simulink model "Automotive_model2"  (R2020b)
settings: Solver=VariableStepAuto  StartTime=0.0  StopTime=97  RelTol=1e-3
undefined symbols (not defined in the file): sigbuilder_block
libraries: simulink x23
(part 2 of 2)

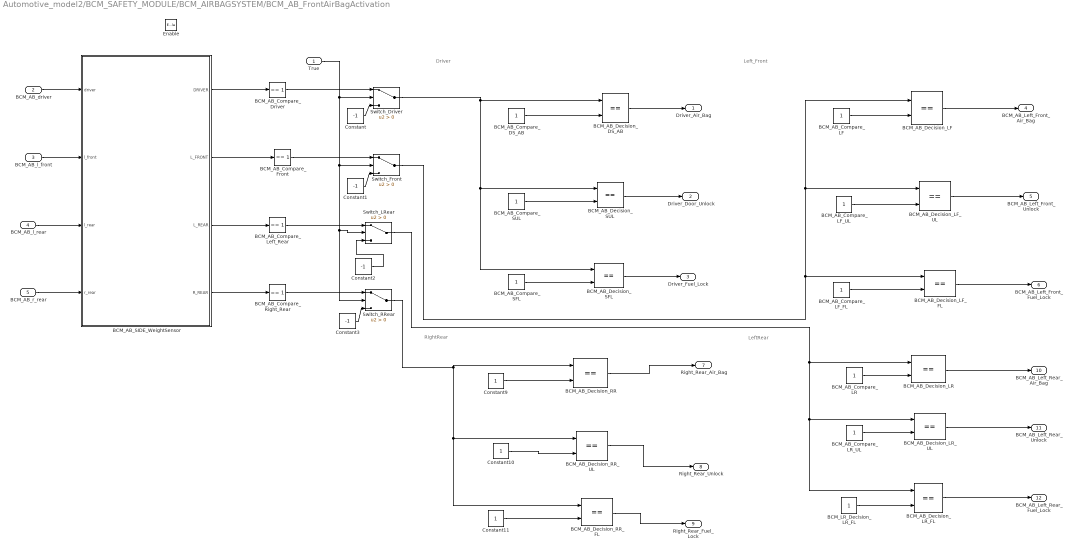
== system Automotive_model2/BCM_SAFETY_MODULE/BCM_AIRBAGSYSTEM/BCM_AB_FrontAirBagActivation ==
  note: RightRear
  note: LeftRear
  note: Left_Front
  note: Driver
  True : Inport
  BCM_AB_driver : Inport  Port=2
  BCM_AB_l_front : Inport  Port=3
  BCM_AB_l_rear : Inport  Port=4
  BCM_AB_r_rear : Inport  Port=5
  Enable : EnablePort
  BCM_AB_Compare_DS_AB : Constant
  BCM_AB_Compare_Driver : simulink/Logic and Bit Operations/Compare To Constant  relop===  const=1  OutDataTypeStr=boolean
  BCM_AB_Compare_Front : simulink/Logic and Bit Operations/Compare To Constant  relop===  const=1  OutDataTypeStr=boolean
  BCM_AB_Compare_LF : Constant
  BCM_AB_Compare_LF_FL : Constant
  BCM_AB_Compare_LF_UL : Constant
  BCM_AB_Compare_LR : Constant
  BCM_AB_Compare_LR_UL : Constant
  BCM_AB_Compare_Left_Rear : simulink/Logic and Bit Operations/Compare To Constant  relop===  const=1  OutDataTypeStr=boolean
  BCM_AB_Compare_Right_Rear : simulink/Logic and Bit Operations/Compare To Constant  relop===  const=1  OutDataTypeStr=boolean
  BCM_AB_Compare_SFL : Constant
  BCM_AB_Compare_SUL : Constant
  BCM_AB_Decision_DS_AB : RelationalOperator  Operator===  OutDataTypeStr=boolean  RndMeth=Simplest
  BCM_AB_Decision_LF : RelationalOperator  Operator===  OutDataTypeStr=boolean  RndMeth=Simplest
  BCM_AB_Decision_LF_FL : RelationalOperator  Operator===  OutDataTypeStr=boolean  RndMeth=Simplest
  BCM_AB_Decision_LF_UL : RelationalOperator  Operator===  OutDataTypeStr=boolean  RndMeth=Simplest
  BCM_AB_Decision_LR : RelationalOperator  Operator===  OutDataTypeStr=boolean  RndMeth=Simplest
  BCM_AB_Decision_LR_FL : RelationalOperator  Operator===  OutDataTypeStr=boolean  RndMeth=Simplest
  BCM_AB_Decision_LR_UL : RelationalOperator  Operator===  OutDataTypeStr=boolean  RndMeth=Simplest
  BCM_AB_Decision_RR : RelationalOperator  Operator===  OutDataTypeStr=boolean  RndMeth=Simplest
  BCM_AB_Decision_RR_FL : RelationalOperator  Operator===  OutDataTypeStr=boolean  RndMeth=Simplest
  BCM_AB_Decision_RR_UL : RelationalOperator  Operator===  OutDataTypeStr=boolean  RndMeth=Simplest
  BCM_AB_Decision_SFL : RelationalOperator  Operator===  OutDataTypeStr=boolean  RndMeth=Simplest
  BCM_AB_Decision_SUL : RelationalOperator  Operator===  OutDataTypeStr=boolean  RndMeth=Simplest
  BCM_AB_SIDE_WeightSensor : MATLAB Function  TreatAsAtomicUnit=on
  BCM_LR_Decision_LR_FL : Constant
  Constant{,1..3} (4 alike) : Constant  Value=-1
  Constant10 : Constant
  Constant11 : Constant
  Constant9 : Constant
  Switch_Driver : Switch  Criteria=u2 > Threshold
  Switch_Front : Switch  Criteria=u2 > Threshold
  Switch_LRear : Switch  Criteria=u2 > Threshold
  Switch_RRear : Switch  Criteria=u2 > Threshold
  Driver_Air_Bag : Outport
  Driver_Door_Unlock : Outport  Port=2
  Driver_Fuel_Lock : Outport  Port=3
  BCM_AB_Left_Front_Air_Bag : Outport  Port=4
  BCM_AB_Left_Front_Unlock : Outport  Port=5
  BCM_AB_Left_Front_Fuel_Lock : Outport  Port=6
  Right_Rear_Air_Bag : Outport  Port=7
  Right_Rear_Unlock : Outport  Port=8
  Right_Rear_Fuel_Lock : Outport  Port=9
  BCM_AB_Left_Rear_Air_Bag : Outport  Port=10
  BCM_AB_Left_Rear_Unlock : Outport  Port=11
  BCM_AB_Left_Rear_Fuel_Lock : Outport  Port=12
  wires:
  BCM_AB_SIDE_WeightSensor/2(L_FRONT) -> BCM_AB_Compare_Front/1
  BCM_AB_SIDE_WeightSensor/1(DRIVER) -> BCM_AB_Compare_Driver/1
  BCM_AB_SIDE_WeightSensor/3(L_REAR) -> BCM_AB_Compare_Left_Rear/1
  BCM_AB_SIDE_WeightSensor/4(R_REAR) -> BCM_AB_Compare_Right_Rear/1
  True/1 -> Switch_RRear/2, Switch_LRear/2, Switch_Front/2, Switch_Driver/2
  BCM_AB_Compare_Driver/1 -> Switch_Driver/1
  BCM_AB_Compare_Front/1 -> Switch_Front/1
  BCM_AB_Compare_Left_Rear/1 -> Switch_LRear/1
  BCM_AB_Compare_Right_Rear/1 -> Switch_RRear/1
  BCM_AB_Compare_SFL/1 -> BCM_AB_Decision_SFL/2
  Switch_Driver/1 -> BCM_AB_Decision_SFL/1, BCM_AB_Decision_SUL/1, BCM_AB_Decision_DS_AB/1
  BCM_AB_Compare_SUL/1 -> BCM_AB_Decision_SUL/2
  BCM_AB_Compare_DS_AB/1 -> BCM_AB_Decision_DS_AB/2
  BCM_AB_Compare_LF_UL/1 -> BCM_AB_Decision_LF_UL/2
  BCM_AB_Compare_LF_FL/1 -> BCM_AB_Decision_LF_FL/2
  Switch_Front/1 -> BCM_AB_Decision_LF/1, BCM_AB_Decision_LF_UL/1, BCM_AB_Decision_LF_FL/1
  BCM_AB_Compare_LF/1 -> BCM_AB_Decision_LF/2
  BCM_AB_Compare_LR_UL/1 -> BCM_AB_Decision_LR_UL/2
  BCM_AB_Compare_LR/1 -> BCM_AB_Decision_LR/2
  Switch_LRear/1 -> BCM_AB_Decision_LR_FL/1, BCM_AB_Decision_LR_UL/1, BCM_AB_Decision_LR/1
  BCM_LR_Decision_LR_FL/1 -> BCM_AB_Decision_LR_FL/2
  Switch_RRear/1 -> BCM_AB_Decision_RR/1, BCM_AB_Decision_RR_FL/1, BCM_AB_Decision_RR_UL/1
  Constant11/1 -> BCM_AB_Decision_RR_FL/2
  Constant10/1 -> BCM_AB_Decision_RR_UL/2
  Constant9/1 -> BCM_AB_Decision_RR/2
  BCM_AB_driver/1 -> BCM_AB_SIDE_WeightSensor/1(driver)
  BCM_AB_l_front/1 -> BCM_AB_SIDE_WeightSensor/2(l_front)
  BCM_AB_l_rear/1 -> BCM_AB_SIDE_WeightSensor/3(l_rear)
  BCM_AB_r_rear/1 -> BCM_AB_SIDE_WeightSensor/4(r_rear)
  BCM_AB_Decision_LF/1 -> BCM_AB_Left_Front_Air_Bag/1
  BCM_AB_Decision_LF_UL/1 -> BCM_AB_Left_Front_Unlock/1
  BCM_AB_Decision_LF_FL/1 -> BCM_AB_Left_Front_Fuel_Lock/1
  BCM_AB_Decision_RR/1 -> Right_Rear_Air_Bag/1
  BCM_AB_Decision_RR_UL/1 -> Right_Rear_Unlock/1
  BCM_AB_Decision_RR_FL/1 -> Right_Rear_Fuel_Lock/1
  BCM_AB_Decision_LR/1 -> BCM_AB_Left_Rear_Air_Bag/1
  BCM_AB_Decision_LR_UL/1 -> BCM_AB_Left_Rear_Unlock/1
  BCM_AB_Decision_LR_FL/1 -> BCM_AB_Left_Rear_Fuel_Lock/1
  BCM_AB_Decision_DS_AB/1 -> Driver_Air_Bag/1
  BCM_AB_Decision_SUL/1 -> Driver_Door_Unlock/1
  BCM_AB_Decision_SFL/1 -> Driver_Fuel_Lock/1
  Constant/1 -> Switch_Driver/3
  Constant1/1 -> Switch_Front/3
  Constant2/1 -> Switch_LRear/3
  Constant3/1 -> Switch_RRear/3

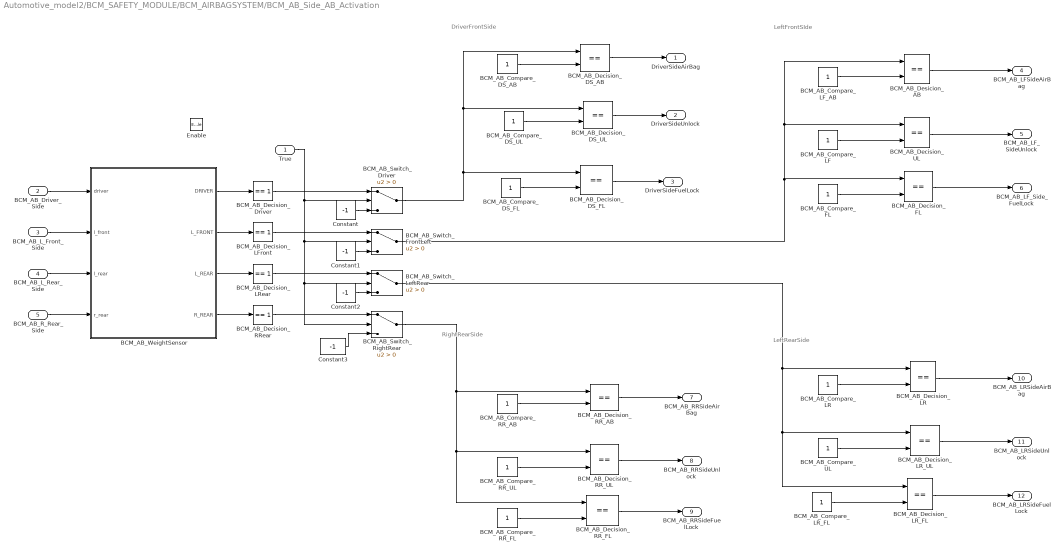
== system Automotive_model2/BCM_SAFETY_MODULE/BCM_AIRBAGSYSTEM/BCM_AB_Side_AB_Activation ==
  note: RightRearSide
  note: LeftRearSide
  note: LeftFrontSIde
  note: DriverFrontSide
  True : Inport
  BCM_AB_Driver_Side : Inport  Port=2
  BCM_AB_L_Front_Side : Inport  Port=3
  BCM_AB_L_Rear_Side : Inport  Port=4
  BCM_AB_R_Rear_Side : Inport  Port=5
  Enable : EnablePort
  BCM_AB_Compare_DS_AB : Constant
  BCM_AB_Compare_DS_FL : Constant
  BCM_AB_Compare_DS_UL : Constant
  BCM_AB_Compare_FL : Constant
  BCM_AB_Compare_LF : Constant
  BCM_AB_Compare_LF_AB : Constant
  BCM_AB_Compare_LR : Constant
  BCM_AB_Compare_LR_FL : Constant
  BCM_AB_Compare_RR_AB : Constant
  BCM_AB_Compare_RR_FL : Constant
  BCM_AB_Compare_RR_UL : Constant
  BCM_AB_Compare_UL : Constant
  BCM_AB_Decision_DS_AB : RelationalOperator  Operator===  OutDataTypeStr=boolean  RndMeth=Simplest
  BCM_AB_Decision_DS_FL : RelationalOperator  Operator===  OutDataTypeStr=boolean  RndMeth=Simplest
  BCM_AB_Decision_DS_UL : RelationalOperator  Operator===  OutDataTypeStr=boolean  RndMeth=Simplest
  BCM_AB_Decision_Driver : simulink/Logic and Bit Operations/Compare To Constant  relop===  const=1  OutDataTypeStr=boolean
  BCM_AB_Decision_FL : RelationalOperator  Operator===  OutDataTypeStr=boolean  RndMeth=Simplest
  BCM_AB_Decision_LFront : simulink/Logic and Bit Operations/Compare To Constant  relop===  const=1  OutDataTypeStr=boolean
  BCM_AB_Decision_LR : RelationalOperator  Operator===  OutDataTypeStr=boolean  RndMeth=Simplest
  BCM_AB_Decision_LR_FL : RelationalOperator  Operator===  OutDataTypeStr=boolean  RndMeth=Simplest
  BCM_AB_Decision_LR_UL : RelationalOperator  Operator===  OutDataTypeStr=boolean  RndMeth=Simplest
  BCM_AB_Decision_LRear : simulink/Logic and Bit Operations/Compare To Constant  relop===  const=1  OutDataTypeStr=boolean
  BCM_AB_Decision_RR_AB : RelationalOperator  Operator===  OutDataTypeStr=boolean  RndMeth=Simplest
  BCM_AB_Decision_RR_FL : RelationalOperator  Operator===  OutDataTypeStr=boolean  RndMeth=Simplest
  BCM_AB_Decision_RR_UL : RelationalOperator  Operator===  OutDataTypeStr=boolean  RndMeth=Simplest
  BCM_AB_Decision_RRear : simulink/Logic and Bit Operations/Compare To Constant  relop===  const=1  OutDataTypeStr=boolean
  BCM_AB_Decision_UL : RelationalOperator  Operator===  OutDataTypeStr=boolean  RndMeth=Simplest
  BCM_AB_Desicion_AB : RelationalOperator  Operator===  OutDataTypeStr=boolean  RndMeth=Simplest
  BCM_AB_Switch_Driver : Switch  Criteria=u2 > Threshold
  BCM_AB_Switch_FrontLeft : Switch  Criteria=u2 > Threshold
  BCM_AB_Switch_LeftRear : Switch  Criteria=u2 > Threshold
  BCM_AB_Switch_RightRear : Switch  Criteria=u2 > Threshold
  BCM_AB_WeightSensor : MATLAB Function  TreatAsAtomicUnit=on
  Constant{,1..3} (4 alike) : Constant  Value=-1
  DriverSideAirBag : Outport
  DriverSideUnlock : Outport  Port=2
  DriverSideFuelLock : Outport  Port=3
  BCM_AB_LFSideAirBag : Outport  Port=4
  BCM_AB_LF_SideUnlock : Outport  Port=5
  BCM_AB_LF_Side_FuelLock : Outport  Port=6
  BCM_AB_RRSideAirBag : Outport  Port=7
  BCM_AB_RRSideUnlock : Outport  Port=8
  BCM_AB_RRSideFuelLock : Outport  Port=9
  BCM_AB_LRSideAirBag : Outport  Port=10
  BCM_AB_LRSideUnlock : Outport  Port=11
  BCM_AB_LRSideFuelLock : Outport  Port=12
  wires:
  BCM_AB_WeightSensor/2(L_FRONT) -> BCM_AB_Decision_LFront/1
  BCM_AB_WeightSensor/3(L_REAR) -> BCM_AB_Decision_LRear/1
  BCM_AB_WeightSensor/4(R_REAR) -> BCM_AB_Decision_RRear/1
  BCM_AB_Decision_LFront/1 -> BCM_AB_Switch_FrontLeft/1
  True/1 -> BCM_AB_Switch_RightRear/2, BCM_AB_Switch_LeftRear/2, BCM_AB_Switch_FrontLeft/2, BCM_AB_Switch_Driver/2
  BCM_AB_WeightSensor/1(DRIVER) -> BCM_AB_Decision_Driver/1
  BCM_AB_Decision_RRear/1 -> BCM_AB_Switch_RightRear/1
  BCM_AB_Decision_LRear/1 -> BCM_AB_Switch_LeftRear/1
  BCM_AB_Decision_Driver/1 -> BCM_AB_Switch_Driver/1
  BCM_AB_Driver_Side/1 -> BCM_AB_WeightSensor/1(driver)
  BCM_AB_R_Rear_Side/1 -> BCM_AB_WeightSensor/4(r_rear)
  BCM_AB_L_Rear_Side/1 -> BCM_AB_WeightSensor/3(l_rear)
  BCM_AB_L_Front_Side/1 -> BCM_AB_WeightSensor/2(l_front)
  BCM_AB_Compare_DS_FL/1 -> BCM_AB_Decision_DS_FL/2
  BCM_AB_Compare_DS_UL/1 -> BCM_AB_Decision_DS_UL/2
  BCM_AB_Compare_DS_AB/1 -> BCM_AB_Decision_DS_AB/2
  BCM_AB_Switch_Driver/1 -> BCM_AB_Decision_DS_AB/1, BCM_AB_Decision_DS_UL/1, BCM_AB_Decision_DS_FL/1
  BCM_AB_Compare_LF/1 -> BCM_AB_Decision_UL/2
  BCM_AB_Compare_LF_AB/1 -> BCM_AB_Desicion_AB/2
  BCM_AB_Compare_FL/1 -> BCM_AB_Decision_FL/2
  BCM_AB_Switch_FrontLeft/1 -> BCM_AB_Desicion_AB/1, BCM_AB_Decision_UL/1, BCM_AB_Decision_FL/1
  BCM_AB_Compare_LR_FL/1 -> BCM_AB_Decision_LR_FL/2
  BCM_AB_Switch_LeftRear/1 -> BCM_AB_Decision_LR/1, BCM_AB_Decision_LR_FL/1, BCM_AB_Decision_LR_UL/1
  BCM_AB_Compare_UL/1 -> BCM_AB_Decision_LR_UL/2
  BCM_AB_Compare_LR/1 -> BCM_AB_Decision_LR/2
  BCM_AB_Compare_RR_FL/1 -> BCM_AB_Decision_RR_FL/2
  BCM_AB_Switch_RightRear/1 -> BCM_AB_Decision_RR_FL/1, BCM_AB_Decision_RR_UL/1, BCM_AB_Decision_RR_AB/1
  BCM_AB_Compare_RR_AB/1 -> BCM_AB_Decision_RR_AB/2
  BCM_AB_Compare_RR_UL/1 -> BCM_AB_Decision_RR_UL/2
  BCM_AB_Decision_DS_AB/1 -> DriverSideAirBag/1
  BCM_AB_Decision_DS_UL/1 -> DriverSideUnlock/1
  BCM_AB_Decision_DS_FL/1 -> DriverSideFuelLock/1
  BCM_AB_Desicion_AB/1 -> BCM_AB_LFSideAirBag/1
  BCM_AB_Decision_UL/1 -> BCM_AB_LF_SideUnlock/1
  BCM_AB_Decision_FL/1 -> BCM_AB_LF_Side_FuelLock/1
  BCM_AB_Decision_RR_AB/1 -> BCM_AB_RRSideAirBag/1
  BCM_AB_Decision_RR_UL/1 -> BCM_AB_RRSideUnlock/1
  BCM_AB_Decision_RR_FL/1 -> BCM_AB_RRSideFuelLock/1
  BCM_AB_Decision_LR/1 -> BCM_AB_LRSideAirBag/1
  BCM_AB_Decision_LR_UL/1 -> BCM_AB_LRSideUnlock/1
  BCM_AB_Decision_LR_FL/1 -> BCM_AB_LRSideFuelLock/1
  Constant/1 -> BCM_AB_Switch_Driver/3
  Constant1/1 -> BCM_AB_Switch_FrontLeft/3
  Constant2/1 -> BCM_AB_Switch_LeftRear/3
  Constant3/1 -> BCM_AB_Switch_RightRear/3

== system Automotive_model2/BCM_SAFETY_MODULE/BCM_Powerwindow_and_Door_operation/BCM_Door_system ==
  DC_Acc : Inport
  DC_iginition : Inport  Port=2
  DC_Door1 : Inport  Port=3
  DC_Door2 : Inport  Port=4
  DC_Door3 : Inport  Port=5
  DC_Door4 : Inport  Port=6
  DC_Antilock : Inport  Port=7
  BCM_Automatic_Door_lock : Subsystem
  BCM_Delay_System_door lock and BCM_interior light subsystem : Subsystem
  Compare To Constant : simulink/Logic and Bit Operations/Compare To Constant  relop=>  const=0  OutDataTypeStr=boolean
  OR1 : Logic  Operator=OR  IconShape=distinctive  AllPortsSameDT=off  OutDataTypeStr=boolean
  Out1 : Outport
  Out2 : Outport  Port=2
  y : Outport  Port=3
  Outport : Outport  Port=4
  wires:
  DC_Door2/1 -> BCM_Delay_System_door lock and BCM_interior light subsystem/2(DC_Door2)
  BCM_Delay_System_door lock and BCM_interior light subsystem/1(Out1) -> Compare To Constant/1
  OR1/1 -> Out2/1
  Compare To Constant/1 -> y/1, OR1/2
  DC_Antilock/1 -> BCM_Delay_System_door lock and BCM_interior light subsystem/5(DC_Antilock)
  BCM_Automatic_Door_lock/1(Out1) -> Out1/1, OR1/1
  DC_Acc/1 -> BCM_Automatic_Door_lock/1(DC_Acc)
  DC_Door3/1 -> BCM_Delay_System_door lock and BCM_interior light subsystem/3(DC_Door3)
  DC_Door4/1 -> BCM_Delay_System_door lock and BCM_interior light subsystem/4(DC_Door4)
  DC_iginition/1 -> BCM_Automatic_Door_lock/2(DC_iginition)
  DC_Door1/1 -> BCM_Delay_System_door lock and BCM_interior light subsystem/1(DC_Door1)
  BCM_Delay_System_door lock and BCM_interior light subsystem/2(Outport) -> Outport/1

== system Automotive_model2/BCM_SAFETY_MODULE/BCM_Powerwindow_and_Door_operation/Front_left_subsystem ==
  lock/unlock : Inport
  In_fl_b : Inport  Port=2
  In_fl_Dc : Inport  Port=3
  object : Inport  Port=4
  Enable : EnablePort
  Display1 : Display
  Switch : Switch  Criteria=u2 ~= 0
  Switch1 : Switch  Criteria=u2 > Threshold
  decision_Box : Stateflow chart  TreatAsAtomicUnit=on
  Outport : Outport
  Outport1 : Outport  Port=2
  wires:
  decision_Box/2(warning) -> Outport/1
  object/1 -> decision_Box/2(data1)
  decision_Box/1(op1) -> Outport1/1, Display1/1
  Switch/1 -> decision_Box/1(data)
  Switch1/1 -> Switch/3
  In_fl_b/1 -> Switch1/3
  In_fl_Dc/1 -> Switch/2, Switch/1, Switch1/1
  lock/unlock/1 -> Switch1/2

== system Automotive_model2/BCM_SAFETY_MODULE/BCM_Powerwindow_and_Door_operation/Rear_right_Subsystem ==
  lock/unlock : Inport
  rear_right_passenger : Inport  Port=2
  rear_right_driver : Inport  Port=3
  object : Inport  Port=4
  Enable : EnablePort
  Chart1 : Stateflow chart  TreatAsAtomicUnit=on
  Display3 : Display
  Switch : Switch  Criteria=u2 ~= 0
  Switch1 : Switch  Criteria=u2 > Threshold
  Outport : Outport
  Outport1 : Outport  Port=2
  wires:
  Chart1/2(warning) -> Outport/1  "ss3"
  object/1 -> Chart1/2(data1)
  Switch/1 -> Chart1/1(data)
  Chart1/1(op1) -> Outport1/1, Display3/1
  Switch1/1 -> Switch/3
  rear_right_passenger/1 -> Switch1/3
  rear_right_driver/1 -> Switch1/1, Switch/2, Switch/1
  lock/unlock/1 -> Switch1/2

== system Automotive_model2/BCM_SAFETY_MODULE/BCM_Powerwindow_and_Door_operation/driver_control_Subsystem ==
  In1 : Inport
  object : Inport  Port=2
  Enable : EnablePort
  Chart : Stateflow chart  TreatAsAtomicUnit=on
  Display4 : Display
  Outport : Outport
  Outport1 : Outport  Port=2
  wires:
  Chart/2(warning) -> Outport/1  "ss4"
  object/1 -> Chart/2(data1)
  In1/1 -> Chart/1(data)
  Chart/1(op1) -> Display4/1, Outport1/1

== system Automotive_model2/BCM_SAFETY_MODULE/BCM_Powerwindow_and_Door_operation/rear_left_Subsystem ==
  lock/unlock : Inport
  In2 : Inport  Port=2
  In3 : Inport  Port=3
  object : Inport  Port=4
  Enable : EnablePort
  Chart : Stateflow chart  TreatAsAtomicUnit=on
  Switch : Switch  Criteria=u2 ~= 0
  Switch1 : Switch  Criteria=u2 > Threshold
  Outport : Outport
  Outport1 : Outport  Port=2
  wires:
  object/1 -> Chart/2(data1)
  Chart/2(warning) -> Outport/1  "ss2"
  Chart/1(op1) -> Outport1/1
  Switch/1 -> Chart/1(data)
  lock/unlock/1 -> Switch1/2
  In2/1 -> Switch1/3
  Switch1/1 -> Switch/3
  In3/1 -> Switch/2, Switch/1, Switch1/1

== system Automotive_model2/BCM_SAFETY_MODULE/BCM_WC_CONTROL/BCM_WC_FR_Automodes ==
  note: Front_Wiper_automodes
  note: Front Wiper modes :
      | In this we are taking 5 modes
      | Low mode for low wiping of windshield
      | Medium mode for Medium speed wiping of windshield
      | High mode for High speed wiping
      | Mist mode for 1x wipe to clear fog and dust from windshield
      | Spray to enable the spray
  BCM_FR_AUTOMODES : Inport
  BCM_FR_AUTOMODE0 : simulink/Logic and Bit Operations/Compare To Constant  relop===  const=0  OutDataTypeStr=boolean
  BCM_FR_AUTOMODE1 : simulink/Logic and Bit Operations/Compare To Constant  relop===  const=1  OutDataTypeStr=boolean
  BCM_FR_AUTOMODE2 : simulink/Logic and Bit Operations/Compare To Constant  relop===  const=2  OutDataTypeStr=boolean
  BCM_FR_AUTOMODE3 : simulink/Logic and Bit Operations/Compare To Constant  relop===  const=3.0  OutDataTypeStr=boolean
  BCM_FR_AUTOMODE4 : simulink/Logic and Bit Operations/Compare To Constant  relop===  const=4  OutDataTypeStr=boolean
  BCM_FR_AUTOMODE5 : simulink/Logic and Bit Operations/Compare To Constant  relop===  const=5  OutDataTypeStr=boolean
  BCM_FR_AUTOMODE_LOWout : Outport
  BCM_FR_AUTOMODE_OFF : Outport  Port=2
  BCM_FR_AUTOMODE_Mediumout : Outport  Port=3
  BCM_FR_AUTOMODE_High : Outport  Port=4
  BCM_FR_AUTOMODE_Spray : Outport  Port=5
  BCM_FR_AUTOMODE_Mist : Outport  Port=6
  wires:
  BCM_FR_AUTOMODE0/1 -> BCM_FR_AUTOMODE_OFF/1
  BCM_FR_AUTOMODES/1 -> BCM_FR_AUTOMODE5/1, BCM_FR_AUTOMODE4/1, BCM_FR_AUTOMODE3/1, BCM_FR_AUTOMODE2/1, BCM_FR_AUTOMODE1/1, BCM_FR_AUTOMODE0/1
  BCM_FR_AUTOMODE4/1 -> BCM_FR_AUTOMODE_Spray/1
  BCM_FR_AUTOMODE5/1 -> BCM_FR_AUTOMODE_Mist/1
  BCM_FR_AUTOMODE2/1 -> BCM_FR_AUTOMODE_Mediumout/1
  BCM_FR_AUTOMODE1/1 -> BCM_FR_AUTOMODE_LOWout/1
  BCM_FR_AUTOMODE3/1 -> BCM_FR_AUTOMODE_High/1

== system Automotive_model2/BCM_SAFETY_MODULE/BCM_WC_CONTROL/BCM_WC_FR_manual ==
  note: FrontWiper_Manual_Control
  note: Manual inputs:
      | If the manual mode is selected, user get the option to vary the speed of wiper manually.
      | Different speed is defined for different ranges.
  BCM_FRW_Manualmode : Inport
  FW_MANUAL : Inport  Port=2
  BCM_FRM_COND : simulink/Logic and Bit Operations/Compare To Constant  relop=>  const=30  OutDataTypeStr=boolean
  BCM_FRM_COND1 : simulink/Logic and Bit Operations/Compare To Constant  relop=<=  const=60  OutDataTypeStr=boolean
  BCM_FRM_COND2 : simulink/Logic and Bit Operations/Compare To Constant  relop=>  const=60  OutDataTypeStr=boolean
  BCM_FRM_COND3 : simulink/Logic and Bit Operations/Compare To Constant  relop=<=  const=100  OutDataTypeStr=boolean
  BCM_FRM_Selection : Switch  Criteria=u2 > Threshold  Threshold=5
  Bw30_60 : Logic  IconShape=distinctive  AllPortsSameDT=off  OutDataTypeStr=boolean
  Bw60_100 : Logic  IconShape=distinctive  AllPortsSameDT=off  OutDataTypeStr=boolean
  Constant : Constant  Value=-1
  LessThan30 : simulink/Logic and Bit Operations/Compare To Constant  relop=<=  const=30  OutDataTypeStr=boolean
  BCM_FRM_Out : Outport
  BCM_FRM_OUT1 : Outport  Port=2
  BCM_FRM_Bw30_60 : Outport  Port=3
  BCM_FRM__Bw60_100 : Outport  Port=4
  wires:
  BCM_FRW_Manualmode/1 -> BCM_FRM_Selection/2
  FW_MANUAL/1 -> BCM_FRM_COND3/1, BCM_FRM_COND2/1, BCM_FRM_COND1/1, BCM_FRM_COND/1, LessThan30/1, BCM_FRM_Selection/1
  BCM_FRM_COND1/1 -> Bw30_60/2
  BCM_FRM_COND3/1 -> Bw60_100/2
  BCM_FRM_COND/1 -> Bw30_60/1
  Bw60_100/1 -> BCM_FRM__Bw60_100/1
  BCM_FRM_COND2/1 -> Bw60_100/1
  BCM_FRM_Selection/1 -> BCM_FRM_Out/1
  LessThan30/1 -> BCM_FRM_OUT1/1
  Bw30_60/1 -> BCM_FRM_Bw30_60/1
  Constant/1 -> BCM_FRM_Selection/3

== system Automotive_model2/BCM_SAFETY_MODULE/BCM_WC_CONTROL/BCM_WC_Rear_windshield ==
  note: REAR_WIPER
  note: Rear Wiper:
      | If WC_BackS is high, Rear wipers are enabled.
      | The wipers only works in low mode.
      | A clock is added for 30 sec delay in wipers.
  BCM_WC_RearWiperINP : Inport
  BCM_WC_StatusINP : Inport  Port=2
  BCM_WC_COMP : simulink/Logic and Bit Operations/Compare To Constant  relop===  const=1  OutDataTypeStr=boolean
  BCM_WC_Conditioncheck : Logic  IconShape=distinctive  AllPortsSameDT=off  OutDataTypeStr=boolean
  BW_OUT : Outport
  wires:
  BCM_WC_COMP/1 -> BW_OUT/1
  BCM_WC_RearWiperINP/1 -> BCM_WC_Conditioncheck/1
  BCM_WC_StatusINP/1 -> BCM_WC_Conditioncheck/2
  BCM_WC_Conditioncheck/1 -> BCM_WC_COMP/1

== system Automotive_model2/BCM_SAFETY_MODULE/TP_Monitoring/IndicateHigh1 ==
  Enable : EnablePort
  Constant : Constant  Value=0
  Out1 : Outport
  wires:
  Constant/1 -> Out1/1

== system Automotive_model2/BCM_SAFETY_MODULE/TP_Monitoring/IndicateHigh2 ==
  Enable : EnablePort
  Constant : Constant  Value=0
  Out1 : Outport
  wires:
  Constant/1 -> Out1/1

== system Automotive_model2/BCM_SAFETY_MODULE/TP_Monitoring/IndicateHigh3 ==
  Enable : EnablePort
  Constant : Constant  Value=0
  Out1 : Outport
  wires:
  Constant/1 -> Out1/1

== system Automotive_model2/BCM_SAFETY_MODULE/TP_Monitoring/IndicateHigh4 ==
  Enable : EnablePort
  Constant : Constant  Value=0
  Out1 : Outport
  wires:
  Constant/1 -> Out1/1

== system Automotive_model2/BCM_SAFETY_MODULE/TP_Monitoring/IndicateLow1 ==
  Enable : EnablePort
  Constant : Constant
  Out1 : Outport
  wires:
  Constant/1 -> Out1/1

== system Automotive_model2/BCM_SAFETY_MODULE/TP_Monitoring/IndicateLow2 ==
  Enable : EnablePort
  Constant : Constant
  Out1 : Outport
  wires:
  Constant/1 -> Out1/1

== system Automotive_model2/BCM_SAFETY_MODULE/TP_Monitoring/IndicateLow3 ==
  Enable : EnablePort
  Constant : Constant
  Out1 : Outport
  wires:
  Constant/1 -> Out1/1

== system Automotive_model2/BCM_SAFETY_MODULE/TP_Monitoring/IndicateLow4 ==
  Enable : EnablePort
  Constant : Constant
  Out1 : Outport
  wires:
  Constant/1 -> Out1/1

== system Automotive_model2/BCM_SAFETY_MODULE/BCM_Powerwindow_and_Door_operation/BCM_Door_system/BCM_Automatic_Door_lock ==
  note: Description:-If equipped, the doors will lock automatically when all doors are closed, the ignition is on). If a vehicle door is unlocked, and then opened and closed, the doors will lock the vehicle speed becomes faster than 13 km/h (8 mph)
  DC_Acc : Inport
  DC_iginition : Inport  Port=2
  AND : Logic  IconShape=distinctive  AllPortsSameDT=off  OutDataTypeStr=boolean
  Constant : Constant
  Display : Display
  Display1 : Display
  Display2 : Display
  If : If  IfExpression=u1>=13  ElseIfExpressions=u1<13  ShowElse=off
  If Action Subsystem : Subsystem  TreatAsAtomicUnit=on
  If Action Subsystem1 : Subsystem  TreatAsAtomicUnit=on
  OR : Logic  Operator=OR  IconShape=distinctive  AllPortsSameDT=off  OutDataTypeStr=boolean
  reset : Constant  Value=0
  Out1 : Outport
  wires:
  If Action Subsystem1/1(Out1) -> OR/2
  If Action Subsystem/1(Out1) -> OR/1
  DC_iginition/1 -> Display/1, If/1
  Constant/1 -> If Action Subsystem/1(In1)
  DC_Acc/1 -> AND/1, Display1/1
  reset/1 -> If Action Subsystem1/1(In1)
  If/2 -> If Action Subsystem1/Action
  If/1 -> If Action Subsystem/Action
  OR/1 -> AND/2
  AND/1 -> Display2/1, Out1/1

== system Automotive_model2/BCM_SAFETY_MODULE/BCM_Powerwindow_and_Door_operation/BCM_Door_system/BCM_Delay_System_door lock and BCM_interior light subsystem ==
  note: Description:-When unlock button is pressed on the power door lock switch while the door is open, a chime will sound three times indicating delayed locking is active. The doors will lock automatically five seconds after all doors are closed. If a door is reopened before that time, the five-second timer will reset when all doors are closed again.
  DC_Door1 : Inport
  DC_Door2 : Inport  Port=2
  DC_Door3 : Inport  Port=3
  DC_Door4 : Inport  Port=4
  DC_Antilock : Inport  Port=5
  AND : Logic  Inputs=5  IconShape=distinctive  AllPortsSameDT=off  OutDataTypeStr=boolean
  AND1 : Logic  Inputs=4  IconShape=distinctive  AllPortsSameDT=off  OutDataTypeStr=boolean
  Add : Sum
  Compare To Constant : simulink/Logic and Bit Operations/Compare To Constant  relop===  const=0  OutDataTypeStr=boolean
  Constant4 : Constant  Value=0
  Constant5 : Constant  Value=0
  Data Type Conversion : DataTypeConversion
  Delay1 : Delay  DelayLength=1
  Display : Display
  Display1 : Display
  Repeating Sequence Stair : simulink/Sources/Repeating Sequence Stair  OutValues=[1 1]  tsamp=-1  OutMin=[]  OutMax=[]  OutDataTypeStr=double  OutputDataTypeScalingMode=double  OutDataType=fixdt(0,8)  ConRadixGroup=Best Precision: Vector-wise  OutScaling=2^-12
  Scope : Scope
  Switch : Switch  Threshold=5
  Switch1 : Switch
  Out1 : Outport
  Outport : Outport  Port=2
  wires:
  Switch1/1 -> Scope/1, Out1/1, Delay1/1, Display/1
  DC_Antilock/1 -> AND/5
  Repeating Sequence Stair/1 -> Switch1/2
  Delay1/1 -> Add/2
  Constant5/1 -> Switch1/3
  Constant4/1 -> Switch/1
  Add/1 -> Switch/2, Switch/3
  Switch/1 -> Switch1/1
  AND/1 -> Data Type Conversion/1
  DC_Door3/1 -> AND/3, AND1/3
  DC_Door4/1 -> AND1/4, AND/4
  AND1/1 -> Compare To Constant/1
  DC_Door1/1 -> AND1/1, AND/1
  DC_Door2/1 -> AND/2, AND1/2
  Compare To Constant/1 -> Outport/1, Display1/1
  Data Type Conversion/1 -> Add/1

== system Automotive_model2/BCM_SAFETY_MODULE/BCM_Powerwindow_and_Door_operation/BCM_Door_system/BCM_Automatic_Door_lock/If Action Subsystem ==
  In1 : Inport
  Action Port : ActionPort  ActionPortLabel=if(u1>=13)
  Out1 : Outport
  wires:
  In1/1 -> Out1/1

== system Automotive_model2/BCM_SAFETY_MODULE/BCM_Powerwindow_and_Door_operation/BCM_Door_system/BCM_Automatic_Door_lock/If Action Subsystem1 ==
  In1 : Inport
  Action Port : ActionPort  ActionPortLabel=elseif(u1<13)
  Out1 : Outport
  wires:
  In1/1 -> Out1/1

== stateflow chart Automotive_model2/BCM_SAFETY_MODULE/BCM_Powerwindow_and_Door_operation/rear_left_Subsystem/Chart ==
  state Normal
    state Start
      entry:
      op1 = 25;
    state second
      entry:
      op1 = 100;
    state PrepareToStop
      entry:
      op1 = 75;
    state Go
      % Green light
      entry:
      op1 = 50;
    (default) -> Start
    Start -> (junction 9)
    (junction 9) -> (junction 6) : after(1,sec)
    PrepareToStop -> second : after(1,sec)
    (junction 6) -> Go
    Go -> PrepareToStop : after(1,sec)
  state Fault
    entry:
    op1 =0;
    state BlinkOn
      % Red light
      entry:
      warning = 1;
    (default) -> BlinkOn
  state block_start
    entry:
  state Normal2
    state state5
      entry:
      op1=0
    state Start1
      entry:
      op1=op1;
    state two
      entry:
      op1 = 0;
    state four3
      entry:
      op1 = 0;
    state three
      entry:
      op1 = 25;
    state three1
      entry:
      op1 = 0;
    state five2
      entry:
      op1=0;
    state five
      entry:
      op1=50;
    state five1
      entry:
      op1=25;
    state four2
      entry:
      op1 = 25;
    state four
      entry:
      op1 = 75;
    state four1
      entry:
      op1 = 50;
    Start1 -> state5 [order 4] : [op1==0]
    (default) -> Start1
    Start1 -> (junction 142) [order 2] : after(1,sec)[op1==25]
    (junction 142) -> four3
    Start1 -> (junction 89) [order 3]
    Start1 -> (junction 103) [order 5]
    Start1 -> (junction 48) [order 1]
    (junction 103) -> (junction 104) : after(1,sec)[op1==50]
    (junction 48) -> (junction 49) : after(1,sec)[op1==100]
    (junction 89) -> (junction 90) : after(1,sec)[op1==75]
    three -> two : after(1,sec)[op1==25]
    (junction 104) -> four2
    (junction 49) -> four
    five -> three : after(1,sec)[op1==50]
    (junction 90) -> four1
    five1 -> three1 : after(1,sec)[op1==25]
    four2 -> five2 : after(1,sec)[op1==25]
    four -> five : after(1,sec)[op1==75]
    four1 -> five1 : after(1,sec)[op1==50]
  block_start -> Fault [order 2] : [data1 ==1]
  (default) -> block_start
  block_start -> Normal2 [order 3] : [data ==-1 && data1==0]
  Normal -> Fault [order 1] : [data1 == 1]
  block_start -> Normal [order 1] : [data ==1 && data1 ==0 ]
  Normal2 -> block_start [order 1] : [data ==1 && data1 ==0]
  Normal -> block_start [order 2] : [data ==-1]
  Fault -> Normal [order 1] : [data1 == 0 && data==1]{warning=0;}
  Fault -> Normal2 [order 2] : [data1 ==0 && data==-1]{warning=0;}
  Normal2 -> Fault [order 2] : [data1==1]
  data: data input; data1 input; op1 output =0; warning output

== stateflow chart Automotive_model2/BCM_SAFETY_MODULE/BCM_Powerwindow_and_Door_operation/driver_control_Subsystem/Chart ==
  state Normal
    state Start
      entry:
      op1 = 25;
    state second
      entry:
      op1 = 100;
    state PrepareToStop
      entry:
      op1 = 75;
    state Go
      % Green light
      entry:
      op1 = 50;
    (default) -> Start
    Start -> (junction 9)
    (junction 9) -> (junction 6) : after(1,sec)
    PrepareToStop -> second : after(1,sec)
    (junction 6) -> Go
    Go -> PrepareToStop : after(1,sec)
  state Fault
    entry:
    op1 =0;
    state BlinkOn
      % Red light
      entry:
      warning = 1;
    (default) -> BlinkOn
  state block_start
    entry:
  state Normal2
    state state5
      entry:
      op1=0
    state Start1
      entry:
      op1=op1;
    state two
      entry:
      op1 = 0;
    state four3
      entry:
      op1 = 0;
    state three
      entry:
      op1 = 25;
    state three1
      entry:
      op1 = 0;
    state five2
      entry:
      op1=0;
    state five
      entry:
      op1=50;
    state five1
      entry:
      op1=25;
    state four2
      entry:
      op1 = 25;
    state four
      entry:
      op1 = 75;
    state four1
      entry:
      op1 = 50;
    Start1 -> state5 [order 4] : [op1==0]
    (default) -> Start1
    Start1 -> (junction 142) [order 2] : after(1,sec)[op1==25]
    (junction 142) -> four3
    Start1 -> (junction 89) [order 3]
    Start1 -> (junction 103) [order 5]
    Start1 -> (junction 48) [order 1]
    (junction 103) -> (junction 104) : after(1,sec)[op1==50]
    (junction 48) -> (junction 49) : after(1,sec)[op1==100]
    (junction 89) -> (junction 90) : after(1,sec)[op1==75]
    three -> two : after(1,sec)[op1==25]
    (junction 104) -> four2
    (junction 49) -> four
    five -> three : after(1,sec)[op1==50]
    (junction 90) -> four1
    five1 -> three1 : after(1,sec)[op1==25]
    four2 -> five2 : after(1,sec)[op1==25]
    four -> five : after(1,sec)[op1==75]
    four1 -> five1 : after(1,sec)[op1==50]
  block_start -> Fault [order 2] : [data1 ==1]
  (default) -> block_start
  block_start -> Normal2 [order 3] : [data ==-1 && data1==0]
  Normal -> Fault [order 1] : [data1 == 1]
  block_start -> Normal [order 1] : [data ==1 && data1 ==0 ]
  Normal2 -> block_start [order 1] : [data ==1 && data1 ==0]
  Normal -> block_start [order 2] : [data ==-1]
  Fault -> Normal [order 1] : [data1 == 0 && data==1]{warning=0;}
  Fault -> Normal2 [order 2] : [data1 ==0 && data==-1]{warning=0;}
  Normal2 -> Fault [order 2] : [data1==1]
  data: data input; data1 input; op1 output =0; warning output

== stateflow chart Automotive_model2/BCM_SAFETY_MODULE/BCM_Powerwindow_and_Door_operation/Front_left_subsystem/decision_Box ==
  state Normal
    state Start
      entry:
      op1 = 25;
    state second
      entry:
      op1 = 100;
    state PrepareToStop
      entry:
      op1 = 75;
    state Go
      % Green light
      entry:
      op1 = 50;
    (default) -> Start
    Start -> (junction 9)
    (junction 9) -> (junction 6) : after(1,sec)
    PrepareToStop -> second : after(1,sec)
    (junction 6) -> Go
    Go -> PrepareToStop : after(1,sec)
  state Fault
    entry:
    op1 =0;
    state BlinkOn
      % Red light
      entry:
      warning = 1;
    (default) -> BlinkOn
  state block_start
    entry:
  state Normal2
    state Start1
      entry:
      op1=op1;
    state two
      entry:
      op1 = 0;
    state three
      entry:
      op1 = 25;
    state five
      entry:
      op1=50;
    state four
      entry:
      op1 = 75;
    (default) -> Start1
    Start1 -> four : after(1,sec)[op1==100]
    three -> two : after(1,sec)[op1==25]
    five -> three : after(1,sec)[op1==50]
    four -> five : after(1,sec)[op1==75]
  block_start -> Fault [order 3] : [data1 ==1 ]
  (default) -> block_start
  block_start -> Normal2 [order 2] : [data ==-1 ]
  Normal -> Fault [order 1] : [data1 == 1]
  block_start -> Normal [order 1] : [data ==1  ]
  Normal2 -> block_start [order 1] : [data ==1 ]
  Normal -> block_start [order 2] : [data == -1]
  Fault -> Normal [order 1] : [data1 == 0 && data==1]{warning=0;}
  Fault -> Normal2 [order 2] : [data==-1]{warning=0;}
  Normal2 -> Fault [order 2] : [data1==1]
  data: data input; data1 input; op1 output =0; warning output

== matlab function Automotive_model2/BCM_SAFETY_MODULE/BCM_AIRBAGSYSTEM/BCM_AB_CheckCrashType/ActivateAirBagSensor ==
  data: SuddenDeceleration input; AirBagSensor output
function AirBagSensor  = fcn(SuddenDeceleration)
if SuddenDeceleration == 1
         %Front airbag active
   AirBagSensor = 1;
else 
   AirBagSensor = 0;   
end

== matlab function Automotive_model2/BCM_SAFETY_MODULE/BCM_AIRBAGSYSTEM/BCM_AB_FrontAirBagActivation/BCM_AB_SIDE_WeightSensor ==
  data: driver input; DRIVER output; l_front input; L_FRONT output; l_rear input; r_rear input; L_REAR output; R_REAR output
function [DRIVER,L_FRONT,L_REAR,R_REAR] = fcn(driver, l_front,l_rear,r_rear)
    if (driver==0 && l_front==0 && l_rear==0 && r_rear==1)      %0001
        DRIVER=0;
        L_FRONT=0;
        L_REAR=0;
        R_REAR=1;
    
    elseif (driver==0 && l_front==0 && l_rear==1 && r_rear==0)
        DRIVER=0;
        L_FRONT=0;
        L_REAR=1;
        R_REAR=0;
    
    elseif (driver==0 && l_front==0 && l_rear==1 && r_rear==1)
        DRIVER=0;
        L_FRONT=0;
        L_REAR=1;
        R_REAR=1;

    elseif (driver==0 && l_front==1 && l_rear==0 && r_rear==0)
        DRIVER=0;
        L_FRONT=1;
        L_REAR=0;
        R_REAR=0;
    
    elseif (driver==0 && l_front==1 && l_rear==0 && r_rear==1)
        DRIVER=0;
        L_FRONT=1;
        L_REAR=0;
        R_REAR=1;
    
    elseif (driver==0 && l_front==1 && l_rear==1 && r_rear==0)
        DRIVER=0;
        L_FRONT=1;
        L_REAR=1;
        R_REAR=0;
    
    elseif (driver==0 && l_front==1 && l_rear==1 && r_rear==1)
        DRIVER=0;
        L_FRONT=1;
        L_REAR=1;
        R_REAR=1;
    
    elseif (driver==1 && l_front==0 && l_rear==0 && r_rear==0)
        DRIVER=1;
        L_FRONT=0;
        L_REAR=0;
        R_REAR=0;
    
    elseif (driver==1 && l_front==0 && l_rear==0 && r_rear==1)
        DRIVER=1;
        L_FRONT=0;
        L_REAR=0;
        R_REAR=1;
    
    elseif (driver==1 && l_front==0 && l_rear==1 && r_rear==0)
        DRIVER=1;
        L_FRONT=0;
        L_REAR=1;
        R_REAR=0;
    
    elseif (driver==1 && l_front==0 && l_rear==1 && r_rear==1)
        DRIVER=1;
        L_FRONT=0;
        L_REAR=1;
        R_REAR=1;
    
    elseif (driver==1 && l_front==1 && l_rear==0 && r_rear==0)
        DRIVER=1;
        L_FRONT=1;
        L_REAR=0;
        R_REAR=0;
    
    elseif (driver==1 && l_front==1 && l_rear==0 && r_rear==1)
        DRIVER=1;
        L_FRONT=1;
        L_REAR=0;
        R_REAR=1;
    
    elseif (driver==1 && l_front==1 && l_rear==1 && r_rear==0)
        DRIVER=1;
        L_FRONT=1;
        L_REAR=1;
        R_REAR=0;
    
    elseif (driver==1 && l_front==1 && l_rear==1 && r_rear==1)
        DRIVER=1;
        L_FRONT=1;
        L_REAR=1;
        R_REAR=1;
    
    else
        DRIVER=0;
        L_FRONT=0;
        L_REAR=0;
        R_REAR=0;
    end

== matlab function Automotive_model2/BCM_SAFETY_MODULE/BCM_AIRBAGSYSTEM/BCM_AB_Side_AB_Activation/BCM_AB_WeightSensor ==
  data: driver input; DRIVER output; l_front input; L_FRONT output; l_rear input; r_rear input; L_REAR output; R_REAR output
function [DRIVER,L_FRONT,L_REAR,R_REAR] = fcn(driver, l_front,l_rear,r_rear)
    if (driver==0 && l_front==0 && l_rear==0 && r_rear==1)      %0001
        DRIVER=0;
        L_FRONT=0;
        L_REAR=0;
        R_REAR=1;
    
    elseif (driver==0 && l_front==0 && l_rear==1 && r_rear==0)
        DRIVER=0;
        L_FRONT=0;
        L_REAR=1;
        R_REAR=0;
    
    elseif (driver==0 && l_front==0 && l_rear==1 && r_rear==1)
        DRIVER=0;
        L_FRONT=0;
        L_REAR=1;
        R_REAR=1;

    elseif (driver==0 && l_front==1 && l_rear==0 && r_rear==0)
        DRIVER=0;
        L_FRONT=1;
        L_REAR=0;
        R_REAR=0;
    
    elseif (driver==0 && l_front==1 && l_rear==0 && r_rear==1)
        DRIVER=0;
        L_FRONT=1;
        L_REAR=0;
        R_REAR=1;
    
    elseif (driver==0 && l_front==1 && l_rear==1 && r_rear==0)
        DRIVER=0;
        L_FRONT=1;
        L_REAR=1;
        R_REAR=0;
    
    elseif (driver==0 && l_front==1 && l_rear==1 && r_rear==1)
        DRIVER=0;
        L_FRONT=1;
        L_REAR=1;
        R_REAR=1;
    
    elseif (driver==1 && l_front==0 && l_rear==0 && r_rear==0)
        DRIVER=1;
        L_FRONT=0;
        L_REAR=0;
        R_REAR=0;
    
    elseif (driver==1 && l_front==0 && l_rear==0 && r_rear==1)
        DRIVER=1;
        L_FRONT=0;
        L_REAR=0;
        R_REAR=1;
    
    elseif (driver==1 && l_front==0 && l_rear==1 && r_rear==0)
        DRIVER=1;
        L_FRONT=0;
        L_REAR=1;
        R_REAR=0;
    
    elseif (driver==1 && l_front==0 && l_rear==1 && r_rear==1)
        DRIVER=1;
        L_FRONT=0;
        L_REAR=1;
        R_REAR=1;
    
    elseif (driver==1 && l_front==1 && l_rear==0 && r_rear==0)
        DRIVER=1;
        L_FRONT=1;
        L_REAR=0;
        R_REAR=0;
    
    elseif (driver==1 && l_front==1 && l_rear==0 && r_rear==1)
        DRIVER=1;
        L_FRONT=1;
        L_REAR=0;
        R_REAR=1;
    
    elseif (driver==1 && l_front==1 && l_rear==1 && r_rear==0)
        DRIVER=1;
        L_FRONT=1;
        L_REAR=1;
        R_REAR=0;
    
    elseif (driver==1 && l_front==1 && l_rear==1 && r_rear==1)
        DRIVER=1;
        L_FRONT=1;
        L_REAR=1;
        R_REAR=1;
    
    else
        DRIVER=0;
        L_FRONT=0;
        L_REAR=0;
        R_REAR=0;
    end

== stateflow chart Automotive_model2/BCM_SAFETY_MODULE/BCM_Powerwindow_and_Door_operation/Rear_right_Subsystem/Chart1 ==
  state Normal
    state Start
      entry:
      op1 = 25;
    state second
      entry:
      op1 = 100;
    state PrepareToStop
      entry:
      op1 = 75;
    state Go
      % Green light
      entry:
      op1 = 50;
    (default) -> Start
    Start -> (junction 9)
    (junction 9) -> (junction 6) : after(1,sec)
    PrepareToStop -> second : after(1,sec)
    (junction 6) -> Go
    Go -> PrepareToStop : after(1,sec)
  state Fault
    entry:
    op1 =0;
    state BlinkOn
      % Red light
      entry:
      warning = 1;
    (default) -> BlinkOn
  state block_start
    entry:
  state Normal2
    state state5
      entry:
      op1=0
    state Start1
      entry:
      op1=op1;
    state two
      entry:
      op1 = 0;
    state four3
      entry:
      op1 = 0;
    state three
      entry:
      op1 = 25;
    state three1
      entry:
      op1 = 0;
    state five2
      entry:
      op1=0;
    state five
      entry:
      op1=50;
    state five1
      entry:
      op1=25;
    state four2
      entry:
      op1 = 25;
    state four
      entry:
      op1 = 75;
    state four1
      entry:
      op1 = 50;
    Start1 -> state5 [order 4] : [op1==0]
    (default) -> Start1
    Start1 -> (junction 142) [order 2] : after(1,sec)[op1==25]
    (junction 142) -> four3
    Start1 -> (junction 89) [order 3]
    Start1 -> (junction 103) [order 5]
    Start1 -> (junction 48) [order 1]
    (junction 103) -> (junction 104) : after(1,sec)[op1==50]
    (junction 48) -> (junction 49) : after(1,sec)[op1==100]
    (junction 89) -> (junction 90) : after(1,sec)[op1==75]
    three -> two : after(1,sec)[op1==25]
    (junction 104) -> four2
    (junction 49) -> four
    five -> three : after(1,sec)[op1==50]
    (junction 90) -> four1
    five1 -> three1 : after(1,sec)[op1==25]
    four2 -> five2 : after(1,sec)[op1==25]
    four -> five : after(1,sec)[op1==75]
    four1 -> five1 : after(1,sec)[op1==50]
  block_start -> Fault [order 2] : [data1 ==1]
  (default) -> block_start
  block_start -> Normal2 [order 3] : [data ==-1 && data1==0]
  Normal -> Fault [order 1] : [data1 == 1]
  block_start -> Normal [order 1] : [data ==1 && data1 ==0 ]
  Normal2 -> block_start [order 1] : [data ==1 && data1 ==0]
  Normal -> block_start [order 2] : [data ==-1]
  Fault -> Normal [order 1] : [data1 == 0 && data==1]{warning=0;}
  Fault -> Normal2 [order 2] : [data1 ==0 && data==-1]{warning=0;}
  Normal2 -> Fault [order 2] : [data1==1]
  data: data input; data1 input; op1 output =0; warning output
